simulink model "TestServo_Computer"  (R2016b)
settings: Solver=ode3  StartTime=0.0  StopTime=inf  FixedStep=0.001  RelTol=1e-3  EnableMultiTasking=on
libraries: amg_usbconverter_n_connect_lib x3, simulink x3
settings Model: Creator=Hi  LastModifiedBy=Wall
settings DataIOCC: LimitDataPoints=on  SaveFormat=Array
settings OptimizationCC: LifeSpan=inf
settings DebuggingCC: SFUnexpectedBacktrackingDiag=warning  SFNoUnconditionalDefaultTransitionDiag=warning  SFExecutionAtInitializationDiag=none
settings HardwareCC: ProdBitPerPointer=32  ProdBitPerSizeT=32  ProdBitPerPtrDiffT=32  ProdLargestAtomicFloat=None  ProdIntDivRoundTo=Undefined  ProdEndianess=Unspecified  ProdWordSize=32  ProdHWDeviceType=32-bit Generic
settings ModelReferenceCC: PropagateSignalLabelsOutOfModel=off
settings GRTTargetCC: TargetLangStandard=C89/C90 (ANSI)  GeneratePreprocessorConditionals=Disable all
settings ConfigComp: CovMetricSettings=dw  CovHtmlReporting=on  CovSaveCumulativeToWorkspaceVar=on  CovSaveSingleToWorkspaceVar=on  CovExternalEMLEnable=off

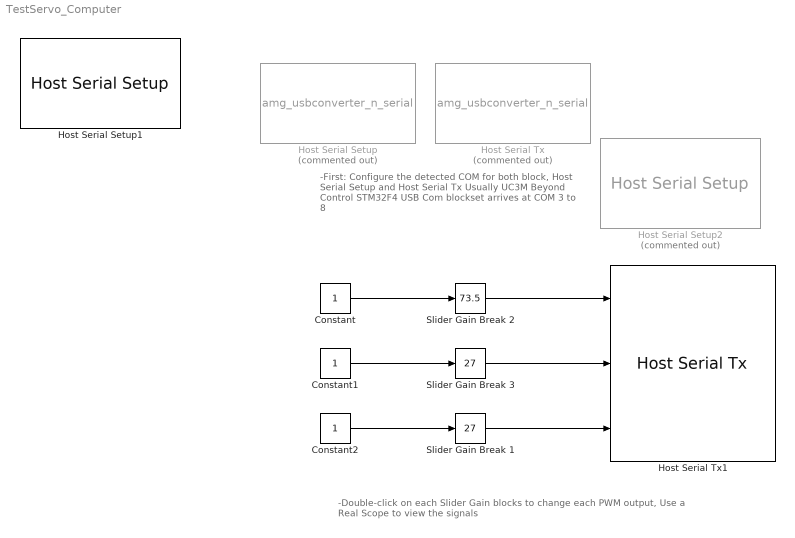
== system TestServo_Computer ==
  note: -First: Configure the detected COM for both block,
      | Host Serial Setup and Host Serial Tx
      | Usually UC3M Beyond Control STM32F4 USB Com
      | blockset arrives at COM 3 to 8
  note: -Double-click on each Slider Gain blocks to change each PWM output,
      | Use a Real Scope to view the signals
  Constant : Constant  OutDataTypeStr=single  SampleTime=-1
  Constant1 : Constant  OutDataTypeStr=single  SampleTime=-1
  Constant2 : Constant  OutDataTypeStr=single  SampleTime=-1
  Host Serial Setup : S-Function  Priority=1  Commented=on  FunctionName=amg_usbconverter_n_serial  Parameters=configuration,port,transfer,baudrate,stopbit,inputtype,outputtype,binheaderarray,binterminatorarray,asciiheader,asciiterminator,bindatalength,packetmode,timeout,sampletime,sampletimestr,blockid  SFunctionDeploymentMode=off  EnableBusSupport=off  mask(amg_usbconverter_n_serial){configuration=Setup, port=COM3, baudrate=10000000, databits=8, parity=None, stopbit=1, flowcontrol=None, advanceoptions=off, rxbuffersize=2048, txbuffersize=2048, transfer=Blocking, timeout=5, packetmode=Binary, binheader='7E 7E', binterminator='03 03', porttype_double=1, porttype_single=0, porttype_int8=1, porttype_uint8=0, porttype_int16=0, porttype_uint16=0, porttype_int32=0, porttype_uint32=0, asciiformat='%d,%f', rx_asciiterminator=CRLF (0x0D 0x0A - "\r\n"), tx_asciiterminator=CR (0x0D - "\r"), inputtype=[0], outputtype=[0], binheaderarray=[2 126  126], binterminatorarray=[2 3  3], bindatalength=0, asciiheader='', asciiterminator=[0], sampletime=inf, sampletimestr=, blockid=HostSerialSetup}
      mask prompts: baudrate "Baud rate (bps)"; databits "Data bits"; stopbit "Stop bit"; flowcontrol "Hardware flow control"; advanceoptions "Advance options"; rxbuffersize "Rx buffer size (bytes)"; txbuffersize "Tx buffer size (bytes)"; timeout "Wait time-out (Seconds)"; packetmode "Packet mode"; binheader "Binary header (example: '7E 7E')"; binterminator "Binary terminator (example: '03 03')"; porttype_double "Number of data port, type DOUBLE"; porttype_single "Number of data port, type SINGLE"; porttype_int8 "Number of data port, type INT8"; porttype_uint8 "Number of data port, type UINT8"; porttype_int16 "Number of data port, type INT16"; porttype_uint16 "Number of data port, type UINT16"; porttype_int32 "Number of data port, type INT32"; porttype_uint32 "Number of data port, type UINT32"; asciiformat "Ascii format"; rx_asciiterminator "End of packet"; tx_asciiterminator "End of packet"; inputtype "Input data type"; outputtype "Output data type"; binheaderarray "Binary header"; binterminatorarray "Binary terminator"; bindatalength "Binary data length"; asciiheader "Ascii header (printf format)"; asciiterminator "Ascii terminator"; sampletime "Sample time (sec)"; sampletimestr "Compiled sample time (sec) in string"
      mask init:
      | amg_usbconverter_n_serial_callback('init');
      mask Help: web(fullfile(waijungdocroot,'amg_usbconverter_n_uart.htm'), '-browser')
      mask TypeOptions configuration: Setup | Tx | Rx
      mask Callback configuration: amg_usbconverter_n_serial_callback('configuration');
      mask TypeOptions port: COM3
      mask Callback port: amg_usbconverter_n_serial_callback('port');
      mask Callback baudrate: amg_usbconverter_n_serial_callback('baudrate');
      mask TypeOptions databits: 8
      mask TypeOptions parity: None
      mask TypeOptions stopbit: 1 | 1.5 | 2
      mask TypeOptions flowcontrol: None | RTS | CTS | RTS/CTS
      mask Callback flowcontrol: amg_usbconverter_n_serial_callback('flowcontrol');
      mask Callback advanceoptions: amg_usbconverter_n_serial_callback('advanceoptions');
      mask TypeOptions rxbuffersize: 16 | 32 | 64 | 128 | 256 | 512 | 1024 | 2048
      mask TypeOptions txbuffersize: 16 | 32 | 64 | 128 | 256 | 512 | 1024 | 2048
      mask TypeOptions transfer: Blocking | Non-Blocking
      mask Callback transfer: amg_usbconverter_n_serial_callback('transfer');
      mask TypeOptions packetmode: Ascii | Binary
      mask Callback packetmode: amg_usbconverter_n_serial_callback('packetmode');
      mask Callback binheader: amg_usbconverter_n_serial_callback('binheader');
      mask Callback binterminator: amg_usbconverter_n_serial_callback('binterminator');
      mask Callback porttype_double: amg_usbconverter_n_serial_callback('porttype');
      mask Callback porttype_single: amg_usbconverter_n_serial_callback('porttype');
      mask Callback porttype_int8: amg_usbconverter_n_serial_callback('porttype');
      mask Callback porttype_uint8: amg_usbconverter_n_serial_callback('porttype');
      mask Callback porttype_int16: amg_usbconverter_n_serial_callback('porttype');
      mask Callback porttype_uint16: amg_usbconverter_n_serial_callback('porttype');
      mask Callback porttype_int32: amg_usbconverter_n_serial_callback('porttype');
      mask Callback porttype_uint32: amg_usbconverter_n_serial_callback('porttype');
      mask Callback asciiformat: amg_usbconverter_n_serial_callback('asciiformat');
      mask TypeOptions rx_asciiterminator: CR (0x0D - "\r") | LF (0x0A - "\n") | CRLF (0x0D 0x0A - "\r\n")
      mask Callback rx_asciiterminator: amg_usbconverter_n_serial_callback('rx_asciiterminator');
      mask TypeOptions tx_asciiterminator: CR (0x0D - "\r") | LF (0x0A - "\n") | CRLF (0x0D 0x0A - "\r\n") | None
      mask Callback tx_asciiterminator: amg_usbconverter_n_serial_callback('tx_asciiterminator');
      mask Callback sampletime: amg_usbconverter_n_serial_callback('sampletime');
      mask Callback sampletimestr: amg_usbconverter_n_serial_callback('sampletimestr');
      mask Callback blockid: amg_usbconverter_n_serial_callback('blockid');
      mask Display: text(0.5, 0.5, 'Port: COM3\nBaud (Bps): 10000000\nFrame: 8-None-1','ver','middle','hor','center');
  Host Serial Setup1 : amg_usbconverter_n_connect_lib/Host Serial Setup  conf=setup  port=<auto>  baudrate=115200  databits=8  parity=None  stopbit=1  flowcontrol=None  transfer=Blocking  timeout=2  packetmode=Binary  initialvalues=[]  binheader='7E 7E'  binterminator='03 03'  porttype_double=0  porttype_single=1  porttype_int8=0  porttype_uint8=0  porttype_int16=0  porttype_uint16=0  porttype_int32=0  porttype_uint32=2  asciiformat='%d %u %x'  rx_asciiterminator="CRLF (0x0D 0x0A - \"\\r\\n\")"  tx_asciiterminator="CRLF (0x0D 0x0A - \"\\r\\n\")"  sampletime=0.02  enablecustomportlabel=off  cinputportlabel=0  coutputportlabel=A  portpinstr=0  blockid=HostSerialSetup1  inputporttype=[]  inputportwidth=[]  inputportlabel={}  outputporttype=[]  outputportwidth=[]  outputportlabel={}  compat=0  optionstring=[]  autoport='COM3'
  Host Serial Setup2 : amg_usbconverter_n_connect_lib/Host Serial Setup  Commented=on  conf=setup  port=<auto>  baudrate=115200  databits=8  parity=None  stopbit=1  flowcontrol=None  transfer=Blocking  timeout=2  packetmode=Binary  initialvalues=[]  binheader='7E 7E'  binterminator='03 03'  porttype_double=0  porttype_single=1  porttype_int8=0  porttype_uint8=0  porttype_int16=0  porttype_uint16=0  porttype_int32=0  porttype_uint32=2  asciiformat='%d %u %x'  rx_asciiterminator="CRLF (0x0D 0x0A - \"\\r\\n\")"  tx_asciiterminator="CRLF (0x0D 0x0A - \"\\r\\n\")"  sampletime=-1  enablecustomportlabel=off  cinputportlabel=0  coutputportlabel=A  portpinstr=0  blockid=HostSerialSetup2  inputporttype=[]  inputportwidth=[]  inputportlabel={}  outputporttype=[]  outputportwidth=[]  outputportlabel={}  compat=0  optionstring="[\"Param1\",\"Param1\"]"  autoport='COM3'
  Host Serial Tx : S-Function  Priority=1  Commented=on  FunctionName=amg_usbconverter_n_serial  Parameters=configuration,port,transfer,baudrate,stopbit,inputtype,outputtype,binheaderarray,binterminatorarray,asciiheader,asciiterminator,bindatalength,packetmode,timeout,sampletime,sampletimestr,blockid  SFunctionDeploymentMode=off  EnableBusSupport=off  mask(amg_usbconverter_n_serial){configuration=Tx, port=<Empty>, baudrate=115200, databits=8, parity=None, stopbit=1, flowcontrol=None, advanceoptions=off, rxbuffersize=2048, txbuffersize=2048, transfer=Blocking, timeout=2, packetmode=Binary, binheader='0E 0E', binterminator='0A 0A', porttype_double=0, porttype_single=2, porttype_int8=0, porttype_uint8=0, porttype_int16=0, porttype_uint16=0, porttype_int32=0, porttype_uint32=0, asciiformat='%d,%f', rx_asciiterminator=CRLF (0x0D 0x0A - "\r\n"), tx_asciiterminator=LF (0x0A - "\n"), inputtype=[2  1 1], outputtype=[0], binheaderarray=[2 14  14], binterminatorarray=[2 10  10], bindatalength=8, asciiheader=['%d,%f' uint8(10)], asciiterminator=[1 10], sampletime=0.01, sampletimestr=, blockid=HostSerialTx}
      mask prompts: baudrate "Baud rate (bps)"; databits "Data bits"; stopbit "Stop bit"; flowcontrol "Hardware flow control"; advanceoptions "Advance options"; rxbuffersize "Rx buffer size (bytes)"; txbuffersize "Tx buffer size (bytes)"; timeout "Wait time-out (Seconds)"; packetmode "Packet mode"; binheader "Binary header (example: '7E 7E')"; binterminator "Binary terminator (example: '03 03')"; porttype_double "Number of data port, type DOUBLE"; porttype_single "Number of data port, type SINGLE"; porttype_int8 "Number of data port, type INT8"; porttype_uint8 "Number of data port, type UINT8"; porttype_int16 "Number of data port, type INT16"; porttype_uint16 "Number of data port, type UINT16"; porttype_int32 "Number of data port, type INT32"; porttype_uint32 "Number of data port, type UINT32"; asciiformat "Ascii format"; rx_asciiterminator "End of packet"; tx_asciiterminator "End of packet"; inputtype "Input data type"; outputtype "Output data type"; binheaderarray "Binary header"; binterminatorarray "Binary terminator"; bindatalength "Binary data length"; asciiheader "Ascii header (printf format)"; asciiterminator "Ascii terminator"; sampletime "Sample time (sec)"; sampletimestr "Compiled sample time (sec) in string"
      mask init:
      | amg_usbconverter_n_serial_callback('init');
      mask Help: web(fullfile(waijungdocroot,'amg_usbconverter_n_uart.htm'), '-browser')
      mask TypeOptions configuration: Setup | Tx | Rx
      mask Callback configuration: amg_usbconverter_n_serial_callback('configuration');
      mask TypeOptions port: COM3 | <Empty>
      mask Callback port: amg_usbconverter_n_serial_callback('port');
      mask Callback baudrate: amg_usbconverter_n_serial_callback('baudrate');
      mask TypeOptions databits: 8
      mask TypeOptions parity: None
      mask TypeOptions stopbit: 1 | 1.5 | 2
      mask TypeOptions flowcontrol: None | RTS | CTS | RTS/CTS
      mask Callback flowcontrol: amg_usbconverter_n_serial_callback('flowcontrol');
      mask Callback advanceoptions: amg_usbconverter_n_serial_callback('advanceoptions');
      mask TypeOptions rxbuffersize: 16 | 32 | 64 | 128 | 256 | 512 | 1024 | 2048
      mask TypeOptions txbuffersize: 16 | 32 | 64 | 128 | 256 | 512 | 1024 | 2048
      mask TypeOptions transfer: Blocking | Non-Blocking
      mask Callback transfer: amg_usbconverter_n_serial_callback('transfer');
      mask TypeOptions packetmode: Ascii | Binary
      mask Callback packetmode: amg_usbconverter_n_serial_callback('packetmode');
      mask Callback binheader: amg_usbconverter_n_serial_callback('binheader');
      mask Callback binterminator: amg_usbconverter_n_serial_callback('binterminator');
      mask Callback porttype_double: amg_usbconverter_n_serial_callback('porttype');
      mask Callback porttype_single: amg_usbconverter_n_serial_callback('porttype');
      mask Callback porttype_int8: amg_usbconverter_n_serial_callback('porttype');
      mask Callback porttype_uint8: amg_usbconverter_n_serial_callback('porttype');
      mask Callback porttype_int16: amg_usbconverter_n_serial_callback('porttype');
      mask Callback porttype_uint16: amg_usbconverter_n_serial_callback('porttype');
      mask Callback porttype_int32: amg_usbconverter_n_serial_callback('porttype');
      mask Callback porttype_uint32: amg_usbconverter_n_serial_callback('porttype');
      mask Callback asciiformat: amg_usbconverter_n_serial_callback('asciiformat');
      mask TypeOptions rx_asciiterminator: CR (0x0D - "\r") | LF (0x0A - "\n") | CRLF (0x0D 0x0A - "\r\n")
      mask Callback rx_asciiterminator: amg_usbconverter_n_serial_callback('rx_asciiterminator');
      mask TypeOptions tx_asciiterminator: CR (0x0D - "\r") | LF (0x0A - "\n") | CRLF (0x0D 0x0A - "\r\n") | None
      mask Callback tx_asciiterminator: amg_usbconverter_n_serial_callback('tx_asciiterminator');
      mask Callback sampletime: amg_usbconverter_n_serial_callback('sampletime');
      mask Callback sampletimestr: amg_usbconverter_n_serial_callback('sampletimestr');
      mask Callback blockid: amg_usbconverter_n_serial_callback('blockid');
      mask Display: text(0.95, 0.5, 'Port: <Empty>\nPacket: Binary\nTransfer: Blocking\nTs (sec): -1','ver','middle','hor','right');port_label('input', 1,'single');port_label('input', 2,'single');
  Host Serial Tx1 : amg_usbconverter_n_connect_lib/Host Serial Tx  conf=tx  port=<auto>  baudrate=115200  databits=8  parity=None  stopbit=1  flowcontrol=None  transfer=Blocking  timeout=2  packetmode=Binary  initialvalues=[]  binheader='0E 0E'  binterminator='0A 0A'  porttype_double=0  porttype_single=3  porttype_int8=0  porttype_uint8=0  porttype_int16=0  porttype_uint16=0  porttype_int32=0  porttype_uint32=0  asciiformat='%d,%f'  rx_asciiterminator="CRLF (0x0D 0x0A - \"\\r\\n\")"  tx_asciiterminator="CRLF (0x0D 0x0A - \"\\r\\n\")"  sampletime=0.002  enablecustomportlabel=off  cinputportlabel=0  coutputportlabel=A  portpinstr=0  blockid=HostSerialTx1  inputporttype=[1 1 1]  inputportwidth=[1 1 1]  inputportlabel={'single','single','single'}  outputporttype=[]  outputportwidth=[]  outputportlabel={}  compat=0  optionstring=[]  autoport='COM3'
  Slider Gain Break 1 : simulink/Math Operations/Slider Gain  low=27  gain=27  high=73.5
  Slider Gain Break 2 : simulink/Math Operations/Slider Gain  low=27  gain=73.5  high=73.5
  Slider Gain Break 3 : simulink/Math Operations/Slider Gain  low=27  gain=27  high=73.5
  wires:
  Constant/1 -> Slider Gain Break 2/1
  Slider Gain Break 2/1 -> Host Serial Tx1/1
  Constant1/1 -> Slider Gain Break 3/1
  Slider Gain Break 3/1 -> Host Serial Tx1/2
  Constant2/1 -> Slider Gain Break 1/1
  Slider Gain Break 1/1 -> Host Serial Tx1/3
